simulink model "invpend"  (R2023b)
settings: Solver=ode45  StartTime=0  StopTime=100  RelTol=1e-3  EnableMultiTasking=on
values from neighbouring files (symbols this model uses):
  A = [0       0             1                0 ... (first row only)    [param1.m]
  B = [0 ... (first row only)    [param1.m]
  C = eye(4)    [param1.m]
  D = zeros(4,1)    [param1.m]
  K = place(A,B,p)    [param1.m]
settings Model: Creator=fukao  LastModifiedBy=fukao
settings SolverCC: AlgebraicLoopSolver=TrustRegion
settings DataIOCC: LimitDataPoints=on  SaveFormat=Array  SignalLoggingSaveFormat=ModelDataLogs  ReturnWorkspaceOutputs=off
settings OptimizationCC: InitFltsAndDblsToZero=on  LifeSpan=inf
settings DebuggingCC: SaveWithParameterizedLinksMsg=none  UnderspecifiedInitializationDetection=Classic  MergeDetectMultiDrivingBlocksExec=none  SignalResolutionControl=TryResolveAllWithWarning  MultiTaskDSMMsg=warning  MultiTaskCondExecSysMsg=none  FcnCallInpInsideContextMsg=warning  UnconnectedInputMsg=warning  UnconnectedOutputMsg=warning  UnconnectedLineMsg=warning  SFUnexpectedBacktrackingDiag=warning  SFNoUnconditionalDefaultTransitionDiag=warning  SFExecutionAtInitializationDiag=none  ArithmeticOperatorsInVariantConditions=warning
settings HardwareCC: ProdBitPerPointer=32  ProdBitPerSizeT=32  ProdBitPerPtrDiffT=32  ProdLargestAtomicFloat=None  ProdIntDivRoundTo=Undefined  ProdEndianess=Unspecified  ProdWordSize=32  ProdHWDeviceType=32-bit Generic  TargetUnknown=on
settings ModelReferenceCC: EnableRefExpFcnMdlSchedulingChecks=on  PropagateSignalLabelsOutOfModel=off
settings CodeAppCC: StateflowObjectComments=on
settings GRTTargetCC: TargetFcnLib=ansi_tfl_tmw.mat  TargetLangStandard=C89/C90 (ANSI)  ParMdlRefBuildCompliant=off  CompOptLevelCompliant=off  ConcurrentExecutionCompliant=off  CombineOutputUpdateFcns=off  MATLABClassNameForMDSCustomization=Simulink.SoftwareTarget.TargetSpecificTriggerConfigurationBase  GRTInterface=on
settings ConfigComp: CovMetricSettings=dw  CovSaveCumulativeToWorkspaceVar=on  CovSaveSingleToWorkspaceVar=on

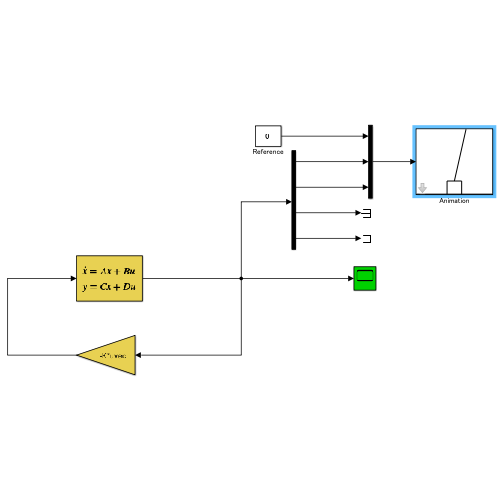
[thumbnail: Simulink's stored preview of the top-level diagram]
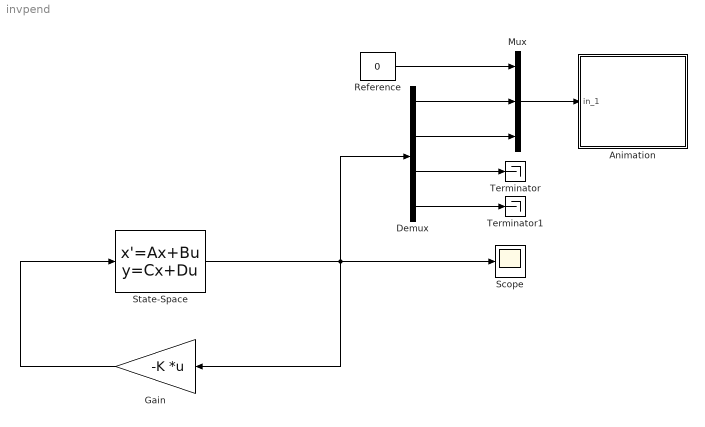
== system invpend ==
  Animation : Subsystem  mask(Pendulum plot){RefBlock=Reference}
      mask prompts: RefBlock "DC reference signal block name:"
      mask help: Pendulum plot
      mask Help: Pendulum animation function using Handle graphics.
      mask Display: plot([-10 10],[0 0],[-2 -2 2 2],[0 1 1 0],[0 3],[1 5])
  Demux : Demux
  Gain : Gain  Gain=-K  Multiplication=Matrix(K*u) (u vector)
  Mux : Mux  Inputs=3
  Reference : Constant  Value=0
  Scope : Scope
  State-Space : StateSpace  A=A  B=B  C=C  D=D  InitialCondition=[5; 0; 0; 0]
  Terminator : Terminator
  Terminator1 : Terminator
  wires:
  State-Space/1 -> Scope/1, Demux/1, Gain/1
  Mux/1 -> Animation/1(in_1)
  Gain/1 -> State-Space/1
  Reference/1 -> Mux/1
  Demux/3 -> Terminator/1
  Demux/4 -> Terminator1/1
  Demux/1 -> Mux/2
  Demux/2 -> Mux/3

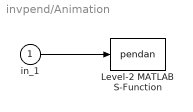
== system invpend/Animation ==
  in_1 : Inport
  Level-2 MATLAB S-Function : M-S-Function  FunctionName=pendan  Parameters=RefBlock
  wires:
  in_1/1 -> Level-2 MATLAB S-Function/1
